simulink subsystem "rxRest"  (R2022a)
settings: Solver=VariableStepAuto  StartTime=0.0  StopTime=10.0  RelTol=1e-3
values from neighbouring files (symbols this model uses):
  bitAlloc = ones(N1, 1) * bitsPerSymbol    [initSefdmModel.m]
  bitsPerFrame = dataNum * N1 * bitsPerSymbol    (= 16256)    [initSefdmModel.m]
  codeLength = actualBlockSize * 24    [initSefdmModel.m]
  codeRate = 1/2    (= 0.5)    [initSefdmModel.m]
  fecLength = 32 / parallelFactor    (= 64)    [initSefdmModel.m]
  infoBitsPerFrame = bitsPerFrame * codeRate - parallel * (constLen - 1)    (= 7366)    [initSefdmModel.m]
  intrlvCol = 1    [initSefdmModel.m]
  intrlvRow = parallel * 2    (= 254)    [initSefdmModel.m]
  noiseVariance = 2/10^(EbNo/10)    (= 0.02)    [initSefdmModel.m]
  useInterleave = 1    [initSefdmModel.m]
libraries: commblkcod2 x1, commblkintrlv2 x1, commdigbbndam3 x1
settings Model: Creator=lsfan  LastModifiedBy=lsfan

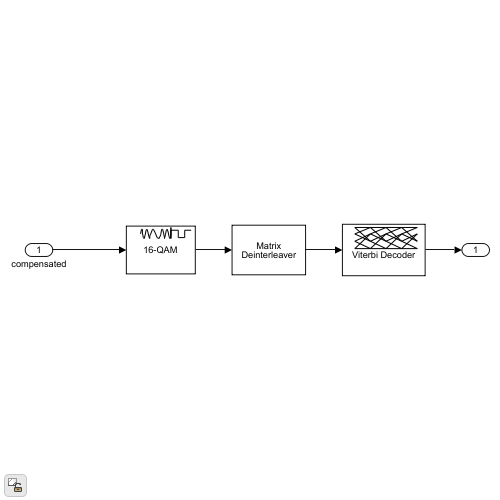
[thumbnail: Simulink's stored preview of the top-level diagram]
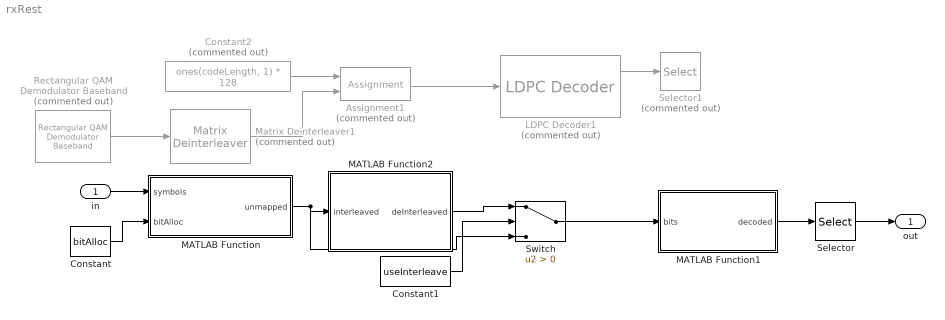
== system rxRest ==
  in : Inport
  Assignment1 : Assignment  Commented=on  DiagnosticForDimensions=Warning  IndexOptions=Index vector (dialog)  Indices=issuedRange  OutputSizes=1
  Constant : Constant  Value=bitAlloc
  Constant1 : Constant  Value=useInterleave
  Constant2 : Constant  Commented=on  Value=ones(codeLength, 1) * 128
  LDPC Decoder1 : commblkcod2/LDPC Decoder  Commented=on  ParityCheckMat=pcmatrix  OutputFmt=Information part  DecisionType=Hard decision  OutputDataType=double  NumIter=ldpcIter  DoParityCheck=off  OutputNumIter=off  OutputFinalChecks=on
      settings: SourceProductBaseCode=CM
  MATLAB Function : MATLAB Function  TreatAsAtomicUnit=on
  MATLAB Function1 : MATLAB Function  TreatAsAtomicUnit=on
  MATLAB Function2 : MATLAB Function  TreatAsAtomicUnit=on
  Matrix Deinterleaver1 : commblkintrlv2/Matrix Deinterleaver  Commented=on  StatePerturbationForJacobian=1.0e-05  Nrows=intrlvRow  Ncols=intrlvCol
      settings: SourceProductBaseCode=CM
  Rectangular QAM Demodulator Baseband : commdigbbndam3/Rectangular QAM Demodulator Baseband  Commented=on  M=M  OutType=Bit  DecType=Approximate log-likelihood ratio  VarSource=Dialog  Variance=noiseVariance  Dec=Gray  Mapping=[0:15]  PowType=Average Power  MinDist=2  AvgPow=1  PeakPow=1  Ph=0  outDtype1=Inherit via internal rule  outDtype2=Inherit via internal rule  derotateFactorWordLen=16  derotateFactorDataTypeStr=Inherit: Same word length as input  derotateFactorLastDataTypeStr=Inherit: Same word length as input  denormFactorWordLen=16  denormFactorDataTypeStr=Inherit: Same word length as input  denormFactorLastDataTypeStr=Inherit: Same word length as input  prodOutWordLen=32  prodOutOverflowMode=Wrap  prodOutRoundingMode=Floor  prodOutOvFlMode=off  prodOutOvFlModeLastStrValue=off  sumWordLen=32
  Selector : Selector  InputPortWidth=bitsPerFrame * codeRate  IndexOptions=Index vector (dialog)  Indices=[1:infoBitsPerFrame]  OutputSizes=1
  Selector1 : Selector  Commented=on  InputPortWidth=dataLength  IndexOptions=Index vector (dialog)  Indices=validRange  OutputSizes=1
  Switch : Switch  Criteria=u2 > Threshold  SaturateOnIntegerOverflow=off  InputSameDT=off
  out : Outport
  wires:
  Assignment1/1 -> LDPC Decoder1/1
  Constant1/1 -> Switch/2
  Selector/1 -> out/1
  MATLAB Function2/1(deInterleaved) -> Switch/1
  LDPC Decoder1/1 -> Selector1/1
  Rectangular QAM Demodulator Baseband/1 -> Matrix Deinterleaver1/1
  Constant2/1 -> Assignment1/1
  Constant/1 -> MATLAB Function/2(bitAlloc)
  Matrix Deinterleaver1/1 -> Assignment1/2
  MATLAB Function1/1(decoded) -> Selector/1
  in/1 -> MATLAB Function/1(symbols)
  Switch/1 -> MATLAB Function1/1(bits)
  MATLAB Function/1(unmapped) -> MATLAB Function2/1(interleaved), Switch/3

== matlab function rxRest/MATLAB Function ==
  data: symbols input; unmapped output; bitAlloc input; N1 parameter
function unmapped = qamdemodFtn(symbols, bitAlloc, N1)
    
    matrix = reshape(symbols, numel(bitAlloc), []);

    temp = zeros(N1 * 4, 16);
    
    current = 0;
    row = 1;
    
    for i = 1:N1
        bit = bitAlloc(i);
        slice = matrix(row, :);
        temp(current+1:current+bit, :) = qamdemod(slice, 2^bit, 'OutputType', 'bit', 'UnitAveragePower', 1);
        current = current + bit;
        row = row + 1;
    end

    unmapped = reshape(temp, [], 1);
    
end

== matlab function rxRest/MATLAB Function1 ==
  data: bits input; decoded output; fecLength parameter; parallel parameter
function decoded = vitdecFTN(bits, fecLength, parallel)

    trellis = poly2trellis(7, [171,133]);
    bits = reshape(bits, parallel, []);
    temp = zeros(parallel,fecLength);
    
    for i = 1:parallel
        slice = bits(i, :);
        temp(i,:) = vitdec(slice, trellis, fecLength,'term', 'hard');
    end

    decoded = reshape(temp, [], 1);
end

== matlab function rxRest/MATLAB Function2 ==
  data: interleaved input; deInterleaved output; parallel parameter; intrlvCol parameter; intrlvRow parameter
function deInterleaved = deInterleave(interleaved, parallel, intrlvCol, intrlvRow)

    interleaved = reshape(interleaved, parallel * 2, 64);
    container = zeros(parallel * 2, 64);
    for i = 1:64
        column = interleaved(:,i);
        temp = circshift(column, -i*4);  % spatial permutation
        container(:, i) = matintrlv(temp, intrlvCol,intrlvRow); % spatial permutation by circular shift
    end

    deInterleaved = reshape(container, [], 1);
